simulink model "analog_tp_1"  (Simulink 5.0)
settings: Solver=ode45  StartTime=0.0  StopTime=0.1  MaxStep=1e-5  RelTol=1e-3
values from neighbouring files (symbols this model uses):
  a = zeros(5, nord+1)    [analog_tp1.m]    (also in analog_tp2.m)
  b = fir1(nr-1,0.5)    [adapt_filter1.m]    (also in adapt_filter2.m; analog_tp1.m = zeros(5, nord+1); analog_tp2.m = zeros(5, nord+1))
libraries: dsparch4 x1
settings Model: Creator=svenhoffmann  LastModifiedBy=svenhoffmann  ExtModeAutoUpdateStatusClock=off  MaxDataPoints=2000

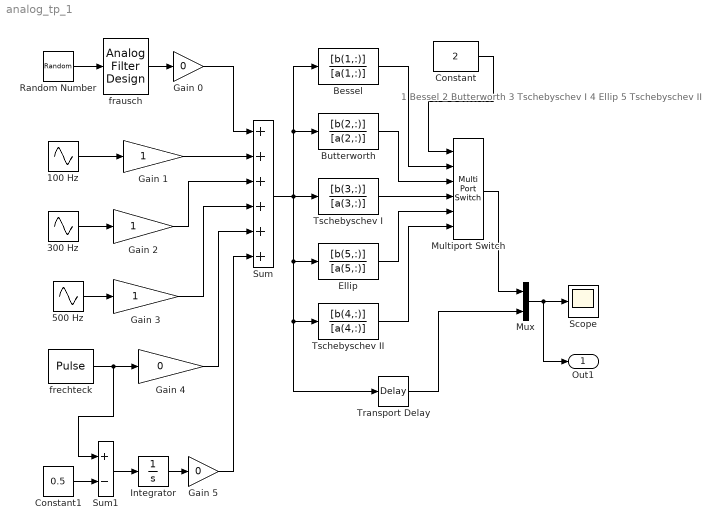
== system analog_tp_1 ==
  note: 1 Bessel
      | 2 Butterworth
      | 3 Tschebyschev I
      | 4 Ellip
      | 5 Tschebyschev II
  100 Hz : Sin  Frequency=2*pi*100  SampleTime=0
  300 Hz : Sin  Amplitude=1/3  Frequency=2*pi*300  SampleTime=0
  500 Hz : Sin  Amplitude=1/5  Frequency=2*pi*500  SampleTime=0
  Bessel : TransferFcn  Numerator=[b(1,:)]  Denominator=[a(1,:)]
  Butterworth : TransferFcn  Numerator=[b(2,:)]  Denominator=[a(2,:)]
  Constant : Constant  Value=2
  Constant1 : Constant  Value=0.5
  Ellip : TransferFcn  Numerator=[b(5,:)]  Denominator=[a(5,:)]
  Gain 0 : Gain  Gain=0  SaturateOnIntegerOverflow=on
  Gain 1 : Gain  SaturateOnIntegerOverflow=on
  Gain 2 : Gain  SaturateOnIntegerOverflow=on
  Gain 3 : Gain  SaturateOnIntegerOverflow=on
  Gain 4 : Gain  Gain=0  SaturateOnIntegerOverflow=on
  Gain 5 : Gain  Gain=0  SaturateOnIntegerOverflow=on
  Integrator : Integrator
  Multiport Switch : MultiPortSwitch  Inputs=5  InputSameDT=on
  Mux : Mux  Inputs=2
  Random Number : RandomNumber  SampleTime=0
  Scope : Scope
      settings: YMin=-1  YMax=1
  Sum : Sum  Inputs=++++++  SaturateOnIntegerOverflow=on  InputSameDT=on
  Sum1 : Sum  Inputs=+-  SaturateOnIntegerOverflow=on  InputSameDT=on
  Transport Delay : TransportDelay  DelayTime=0.9e-3
  Tschebyschev I : TransferFcn  Numerator=[b(3,:)]  Denominator=[a(3,:)]
  Tschebyschev II : TransferFcn  Numerator=[b(4,:)]  Denominator=[a(4,:)]
  frausch : dsparch4/Analog Filter Design  method=Butterworth  filttype=Lowpass  N=8  Wlo=2*pi*500  Whi=80  Rp=2  Rs=40
  frechteck : DiscretePulseGenerator  PulseType=Time based  Period=1/100  PulseWidth=50
  Out1 : Outport
  wires:
  Random Number/1 -> frausch/1
  100 Hz/1 -> Gain 1/1
  300 Hz/1 -> Gain 2/1
  500 Hz/1 -> Gain 3/1
  Gain 0/1 -> Sum/1
  Gain 1/1 -> Sum/2
  Gain 2/1 -> Sum/3
  Gain 3/1 -> Sum/4
  Sum/1 -> Butterworth/1, Bessel/1, Tschebyschev I/1, Transport Delay/1, Tschebyschev II/1, Ellip/1
  Bessel/1 -> Multiport Switch/2
  Butterworth/1 -> Multiport Switch/3
  Tschebyschev I/1 -> Multiport Switch/4
  Ellip/1 -> Multiport Switch/5
  Tschebyschev II/1 -> Multiport Switch/6
  Constant/1 -> Multiport Switch/1
  Mux/1 -> Scope/1, Out1/1
  Multiport Switch/1 -> Mux/1
  Transport Delay/1 -> Mux/2
  frausch/1 -> Gain 0/1
  frechteck/1 -> Gain 4/1, Sum1/1
  Integrator/1 -> Gain 5/1
  Sum1/1 -> Integrator/1
  Constant1/1 -> Sum1/2
  Gain 4/1 -> Sum/5
  Gain 5/1 -> Sum/6
